simulink model "pdl_linear_hw3n"  (R2017a)
settings: Solver=FixedStepAuto  StartTime=0.0  StopTime=duration  FixedStep=Ts  RelTol=1e-3
values from neighbouring files (symbols this model uses):
  A_a = [A E*Cw; zeros(2,4) Aw]    [pendulum_hw3linear.m]
  B_a = [B; zeros(2,1)]    [pendulum_hw3linear.m]
  C_a = [C zeros(2,2)]    [pendulum_hw3linear.m]
  E_a = [zeros(4,2); Bw]    [pendulum_hw3linear.m]
  f_p = 1e-4    (= 0.0001)    [pendulum_hw3linear.m]    (also in pendulum_hw3nonlinear.m)
  K = lqr(A_a,B_a,Q,R)    [pendulum_hw3linear.m]    (also in pendulum_hw3nonlinear.m = lqr(A,B,Q,R))
  m_p = 1e-7    (= 1e-07)    [pendulum_hw3linear.m]    (also in pendulum_hw3nonlinear.m)
  Nbar = -pinv(B_a)*A_a*pinv(Cn)+K*pinv(Cn)    [pendulum_hw3linear.m]    (also in pendulum_hw3nonlinear.m = -pinv(B)*A*pinv(Cn)+K*pinv(Cn))
  Q_k = diag([1 1])    [pendulum_hw3linear.m]    (also in pendulum_hw3nonlinear.m)
  R_k = 1e-4*diag([1 1])    [pendulum_hw3linear.m]    (also in pendulum_hw3nonlinear.m)
  Ts = 0.001    [pendulum_hw3linear.m]    (also in pendulum_hw3nonlinear.m)
  w_p = 10    [pendulum_hw3linear.m]    (also in pendulum_hw3nonlinear.m)
  X_0 = [0;0*pi/180;0;0;0;0]    [pendulum_hw3linear.m]    (also in pendulum_hw3nonlinear.m = [0;0*pi/180;0;0])
undefined symbols (not defined in the file or in its folder): Delta, Gamma, Phi
libraries: simulink x3
settings Model: Creator=Salmon  LastModifiedBy=Salmon

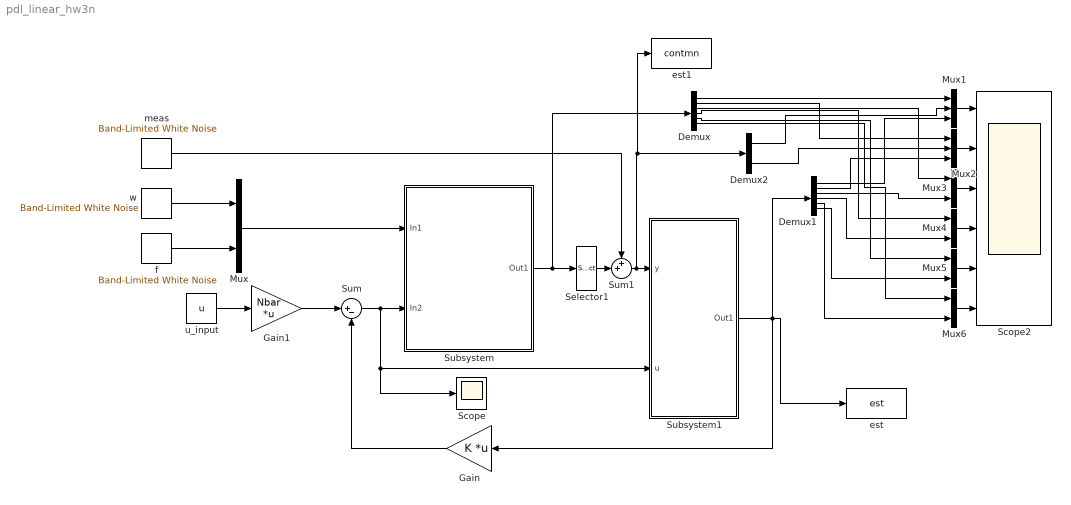
== system pdl_linear_hw3n ==
  Demux : Demux  Outputs=6
  Demux1 : Demux  Outputs=6
  Demux2 : Demux  Outputs=2
  Gain : Gain  Gain=K  Multiplication=Matrix(K*u)
  Gain1 : Gain  Gain=Nbar  Multiplication=Matrix(K*u)
  Mux{,3..6} (5 alike) : Mux  Inputs=2
  Mux1 : Mux  Inputs=3
  Mux2 : Mux  Inputs=3
  Scope : Scope
  Scope2 : Scope  NumInputPorts=6
  Selector1 : Selector  InputPortWidth=6  IndexOptions=Index vector (dialog)  Indices=[1 2]  OutputSizes=1
  Subsystem : Subsystem
  Subsystem1 : Subsystem
  Sum : Sum  Inputs=|+-
  Sum1 : Sum  Inputs=++|
  est : ToWorkspace  VariableName=est  SaveFormat=Structure With Time  SampleTime=Ts
  est1 : ToWorkspace  VariableName=contmn  SaveFormat=Structure With Time  SampleTime=Ts
  f : simulink/Sources/Band-Limited White Noise  Cov=[f_p]  Ts=Ts  seed=[23341]
  meas : simulink/Sources/Band-Limited White Noise  Cov=[m_p,m_p]  Ts=Ts  seed=[123,23341]
  u_input : Constant  Value=u
  w : simulink/Sources/Band-Limited White Noise  Cov=[w_p]  Ts=Ts  seed=[23341]
  wires:
  w/1 -> Mux/1
  f/1 -> Mux/2
  Mux/1 -> Subsystem/1(In1)
  u_input/1 -> Gain1/1
  Subsystem/1(Out1) -> Selector1/1, Demux/1
  Sum/1 -> Subsystem1/2(u), Scope/1, Subsystem/2(In2)
  Gain/1 -> Sum/2
  Gain1/1 -> Sum/1
  Demux/1 -> Mux1/1
  Demux/2 -> Mux2/1
  Demux/3 -> Mux3/1
  Demux/4 -> Mux4/1
  Demux/5 -> Mux5/1
  Demux/6 -> Mux6/1
  Selector1/1 -> Sum1/2
  Demux1/1 -> Mux1/3
  Subsystem1/1(Out1) -> est/1, Gain/1, Demux1/1
  Demux1/3 -> Mux3/2
  Demux1/2 -> Mux2/3
  Demux1/4 -> Mux4/2
  Demux1/5 -> Mux6/2
  Demux1/6 -> Mux5/2
  meas/1 -> Sum1/1
  Demux2/1 -> Mux1/2
  Sum1/1 -> est1/1, Demux2/1, Subsystem1/1(y)
  Demux2/2 -> Mux2/2
  Mux1/1 -> Scope2/1
  Mux2/1 -> Scope2/2
  Mux3/1 -> Scope2/3
  Mux4/1 -> Scope2/4
  Mux5/1 -> Scope2/5
  Mux6/1 -> Scope2/6

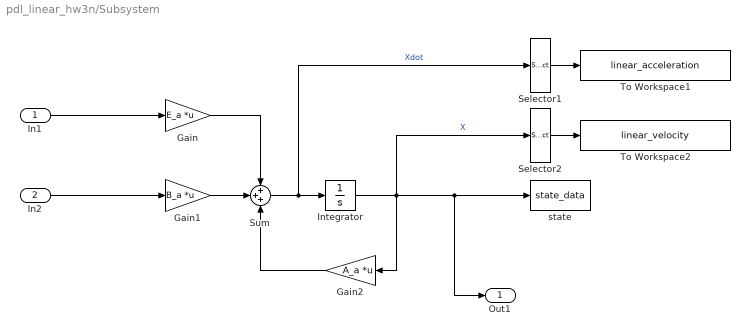
== system pdl_linear_hw3n/Subsystem ==
  In1 : Inport
  In2 : Inport  Port=2
  Gain : Gain  Gain=E_a  Multiplication=Matrix(K*u)
  Gain1 : Gain  Gain=B_a  Multiplication=Matrix(K*u)
  Gain2 : Gain  Gain=A_a  Multiplication=Matrix(K*u)
  Integrator : Integrator  InitialCondition=X_0
  Selector1 : Selector  InputPortWidth=6  IndexOptions=Index vector (dialog)  Indices=[3]  OutputSizes=1
  Selector2 : Selector  InputPortWidth=6  IndexOptions=Index vector (dialog)  Indices=[3]  OutputSizes=1
  Sum : Sum  Inputs=+++
  To Workspace1 : ToWorkspace  VariableName=linear_acceleration  SaveFormat=Structure With Time  SampleTime=-1
  To Workspace2 : ToWorkspace  VariableName=linear_velocity  SaveFormat=Structure With Time  SampleTime=-1
  state : ToWorkspace  VariableName=state_data  SaveFormat=Structure With Time  SampleTime=Ts
  Out1 : Outport
  wires:
  In1/1 -> Gain/1
  Gain/1 -> Sum/1
  Gain1/1 -> Sum/2
  Selector2/1 -> To Workspace2/1
  Selector1/1 -> To Workspace1/1
  Gain2/1 -> Sum/3
  In2/1 -> Gain1/1
  Integrator/1 -> Gain2/1, Selector2/1, Out1/1, state/1  "X"
  Sum/1 -> Integrator/1, Selector1/1  "Xdot"

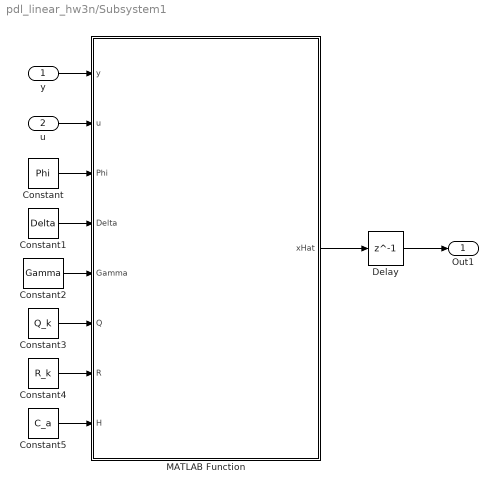
== system pdl_linear_hw3n/Subsystem1 ==
  y : Inport
  u : Inport  Port=2
  Constant : Constant  Value=Phi
  Constant1 : Constant  Value=Delta
  Constant2 : Constant  Value=Gamma
  Constant3 : Constant  Value=Q_k
  Constant4 : Constant  Value=R_k
  Constant5 : Constant  Value=C_a
  Delay : Delay  DelayLength=1  InitialCondition=0
  MATLAB Function : MATLAB Function  TreatAsAtomicUnit=on
  Out1 : Outport
  wires:
  y/1 -> MATLAB Function/1(y)
  MATLAB Function/1(xHat) -> Delay/1
  u/1 -> MATLAB Function/2(u)
  Constant/1 -> MATLAB Function/3(Phi)
  Constant1/1 -> MATLAB Function/4(Delta)
  Constant3/1 -> MATLAB Function/6(Q)
  Constant2/1 -> MATLAB Function/5(Gamma)
  Constant4/1 -> MATLAB Function/7(R)
  Constant5/1 -> MATLAB Function/8(H)
  Delay/1 -> Out1/1

== matlab function pdl_linear_hw3n/Subsystem1/MATLAB Function ==
  data: y input; u input; xHat output; Phi input; Delta input; Gamma input; Q input; R input; H input
function xHat = fcn(y,u,Phi,Delta,Gamma,Q,R,H)

persistent Pbar xbar

% init. Pbar xbar
if isempty(Pbar)
    Pbar = 1e-6*eye(6);
end

if isempty(xbar)
    xbar = zeros(6,1);
end

% 1. Kalman gain
K = Pbar*H'*[H*Pbar*H'+R]^(-1);

% 2. state est. update
xHat = xbar + K*[y-H*xbar];

% 3. error covariance update
Phat = [eye(6)-K*H]*Pbar*[eye(6)-K*H]'+K*R*K';

% 4. state est. propagation
xbar = Phi*xHat+Delta*u;

% 5. error covariance propagation
Pbar = Phi*Phat*Phi'+Gamma*Q*Gamma';
